simulink model "CSAD_Thrust_simulation"  (R2015a)
settings: Solver=ode3  StartTime=0.0  StopTime=350  FixedStep=0.01  MaxStep=10.0  RelTol=1e-3
values from neighbouring files (symbols this model uses):
  C = [C1;C2;C3]    [Spange_init.m]
  D = 3.0/100    (= 0.03)    [Spange_init.m]
  eps_c = 5    [Spange_init.m]
  epsilon = 0.5    [Spange_init.m]
  hd = c2d(H1,0.1,'foh')    [Spange_init.m]
  hd2 = c2d(H2,0.01,'zoh')    [Spange_init.m]
  I_s = 0.05    [Spange_init.m]
  k_cc = 1    [Spange_init.m]
  K_omega = 0.3    [Spange_init.m]
  K_q1f = 0.0113    [Spange_init.m]
  K_q1r = K_q1f    (= 0.0113)    [Spange_init.m]
  K_q2f = 0.0117    [Spange_init.m]
  K_q2r = K_q2f    (= 0.0117)    [Spange_init.m]
  K_q3f = 0.0113    [Spange_init.m]
  K_q3r = K_q3f    (= 0.0113)    [Spange_init.m]
  K_T1f = 0.3763    [Spange_init.m]
  K_T1r = K_T1f    (= 0.3763)    [Spange_init.m]
  K_T2f = 0.3901    [Spange_init.m]
  K_T2r = K_T2f    (= 0.3901)    [Spange_init.m]
  K_T3f = 0.3776    [Spange_init.m]
  K_T3r = K_T3f    (= 0.3776)    [Spange_init.m]
  Kp = 0.3    [Spange_init.m]
  Max_Acceleration = 2    [Spange_init.m]
  Max_rotation = 12*sqrt(lambda)    [Spange_init.m]
  Max_thrust = 1.5034    [Spange_init.m]
  Min_thrust = -0.85    [Spange_init.m]
  n_c = 5    [Spange_init.m]
  n_max = 64.6    [Spange_init.m]
  p_cc = 0.5    [Spange_init.m]
  Q_f0 = 0.3    [Spange_init.m]
  r_cc = 4    [Spange_init.m]
  Rho = Rho_m    (= 1000)    [Spange_init.m]
  tc = [u(1),u(2),u(3)]'    [Spange_thrustallocationQuadratic_mode1.m]    (also in Spange_thrustallocationQuadratic_mode2.m; Spange_thrustallocationQuadratic_mode3.m; Spange_thrustallocationQuadratic_mode4.m)
  Thruster_control = 1    [Spange_init.m]
undefined symbols (not defined in the file or in its folder): K_q4f, K_q4r, K_q5f, K_q5r, K_q6f, K_q6r, K_T4f, K_T4r, K_T5f, K_T5r, K_T6f, K_T6r, Thrust_algorithm, Thruster, Thruster_lock
libraries: simulink x6, simulink_extras x3
(part 1 of 2)
settings Model: CovModelRefEnable=off  Creator=Preben  LastModifiedBy=Preben
settings SolverCC: AlgebraicLoopSolver=LineSearch
settings DataIOCC: SaveFormat=Dataset
settings HardwareCC: ProdBitPerPointer=64  ProdLargestAtomicFloat=Float  ProdIntDivRoundTo=Zero  ProdEndianess=LittleEndian  ProdHWDeviceType=Specified

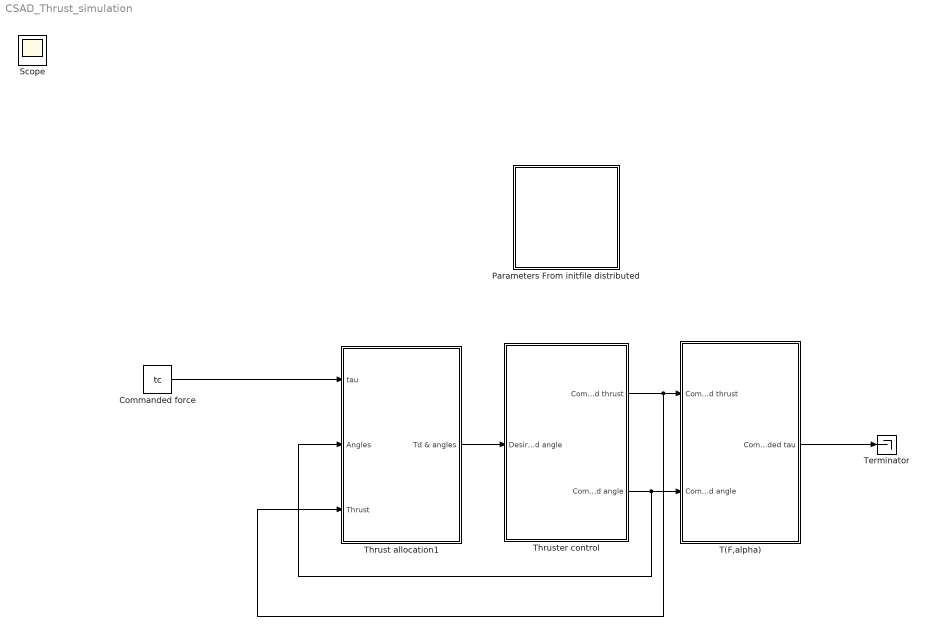
== system CSAD_Thrust_simulation ==
  Commanded force : Constant  Value=tc
  "Parameters From initfile distributed " : Subsystem
  T(F,alpha) : Subsystem
  Terminator : Terminator
  Thrust allocation1 : Subsystem
  "Thruster control " : Subsystem
  Scope : Scope
      settings: YMin=-10  YMax=10  SaveName=ScopeData2
  wires:
  "Thruster control "/2(Commanded angle) -> T(F,alpha)/2(Commanded angle), Thrust allocation1/2(Angles)
  Thrust allocation1/1(Td & angles) -> "Thruster control "/1("Desired thrust and angle ")
  "Thruster control "/1("Commanded thrust ") -> Thrust allocation1/3(Thrust), T(F,alpha)/1(Commanded thrust)
  T(F,alpha)/1(Commanded tau) -> Terminator/1
  Commanded force/1 -> Thrust allocation1/1(tau)

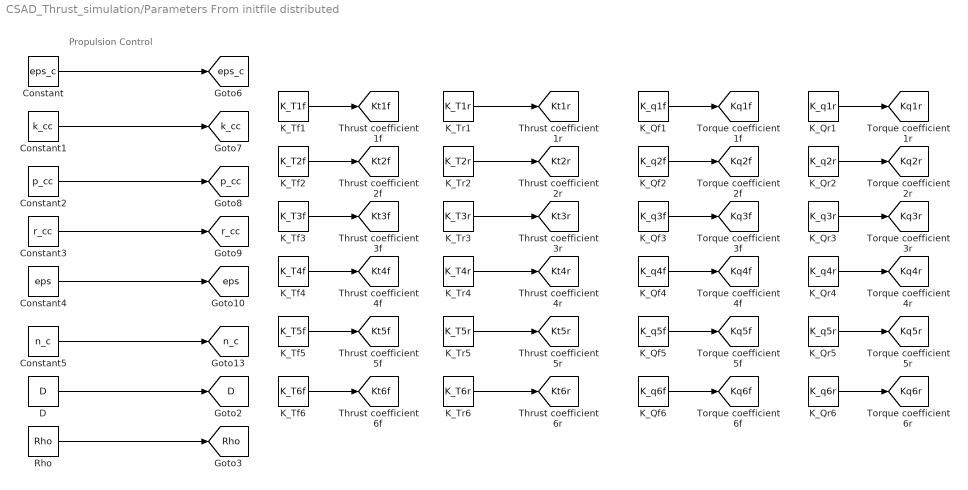
== system CSAD_Thrust_simulation/Parameters From initfile distributed  ==
  note: Propulsion Control
  Constant : Constant  Value=eps_c
  Constant1 : Constant  Value=k_cc
  Constant2 : Constant  Value=p_cc
  Constant3 : Constant  Value=r_cc
  Constant4 : Constant  Value=eps
  Constant5 : Constant  Value=n_c
  D : Constant  Value=D
  K_Qf1 : Constant  Value=K_q1f
  K_Qf2 : Constant  Value=K_q2f
  K_Qf3 : Constant  Value=K_q3f
  K_Qf4 : Constant  Value=K_q4f
  K_Qf5 : Constant  Value=K_q5f
  K_Qf6 : Constant  Value=K_q6f
  K_Qr1 : Constant  Value=K_q1r
  K_Qr2 : Constant  Value=K_q2r
  K_Qr3 : Constant  Value=K_q3r
  K_Qr4 : Constant  Value=K_q4r
  K_Qr5 : Constant  Value=K_q5r
  K_Qr6 : Constant  Value=K_q6r
  K_Tf1 : Constant  Value=K_T1f
  K_Tf2 : Constant  Value=K_T2f
  K_Tf3 : Constant  Value=K_T3f
  K_Tf4 : Constant  Value=K_T4f
  K_Tf5 : Constant  Value=K_T5f
  K_Tf6 : Constant  Value=K_T6f
  K_Tr1 : Constant  Value=K_T1r
  K_Tr2 : Constant  Value=K_T2r
  K_Tr3 : Constant  Value=K_T3r
  K_Tr4 : Constant  Value=K_T4r
  K_Tr5 : Constant  Value=K_T5r
  K_Tr6 : Constant  Value=K_T6r
  Rho : Constant  Value=Rho
  tag scope: D=global, Kq1f=global, Kq1r=global, Kq2f=global, Kq2r=global, Kq3f=global, Kq3r=global, Kq4f=global, Kq4r=global, Kq5f=global, Kq5r=global, Kq6f=global, Kq6r=global, Kt1f=global, Kt1r=global, Kt2f=global, Kt2r=global, Kt3f=global, Kt3r=global, Kt4f=global, Kt4r=global, Kt5f=global, Kt5r=global, Kt6f=global, Kt6r=global, Rho=global, eps=global, eps_c=global, k_cc=global, n_c=global, p_cc=global, r_cc=global
  wires:
  D/1 -> [D]
  Rho/1 -> [Rho]
  Constant/1 -> [eps_c]
  Constant1/1 -> [k_cc]
  Constant2/1 -> [p_cc]
  Constant3/1 -> [r_cc]
  Constant4/1 -> [eps]
  Constant5/1 -> [n_c]
  K_Tf1/1 -> [Kt1f]
  K_Tf6/1 -> [Kt6f]
  K_Tf5/1 -> [Kt5f]
  K_Tf4/1 -> [Kt4f]
  K_Tf3/1 -> [Kt3f]
  K_Tf2/1 -> [Kt2f]
  K_Tr1/1 -> [Kt1r]
  K_Tr6/1 -> [Kt6r]
  K_Tr5/1 -> [Kt5r]
  K_Tr4/1 -> [Kt4r]
  K_Tr2/1 -> [Kt2r]
  K_Tr3/1 -> [Kt3r]
  K_Qf1/1 -> [Kq1f]
  K_Qf2/1 -> [Kq2f]
  K_Qf3/1 -> [Kq3f]
  K_Qf4/1 -> [Kq4f]
  K_Qf5/1 -> [Kq5f]
  K_Qf6/1 -> [Kq6f]
  K_Qr1/1 -> [Kq1r]
  K_Qr2/1 -> [Kq2r]
  K_Qr3/1 -> [Kq3r]
  K_Qr4/1 -> [Kq4r]
  K_Qr5/1 -> [Kq5r]
  K_Qr6/1 -> [Kq6r]

== system CSAD_Thrust_simulation/T(F,alpha) ==
  Commanded thrust : Inport
  Commanded angle : Inport  Port=2
  MATLAB Function : MATLAB Function  TreatAsAtomicUnit=on
  Radians to Degrees : simulink_extras/Transformations/Radians to Degrees
  X-position Thruster : Constant  Value=[Thruster.T1(1) Thruster.T2(1) Thruster.T3(1) Thruster.T4(1) Thruster.T5(1) Thruster.T6(1)]
  Y-position Thruster : Constant  Value=[Thruster.T1(2) Thruster.T2(2) Thruster.T3(2) Thruster.T4(2) Thruster.T5(2) Thruster.T6(2)]
  Commanded tau : Outport
  wires:
  Commanded angle/1 -> Radians to Degrees/1
  X-position Thruster/1 -> MATLAB Function/3(PosX)
  Y-position Thruster/1 -> MATLAB Function/4(PosY)
  MATLAB Function/1(actual_tau) -> Commanded tau/1
  Commanded thrust/1 -> MATLAB Function/1(thrust_actual)
  Radians to Degrees/1 -> MATLAB Function/2(alpha_actual)

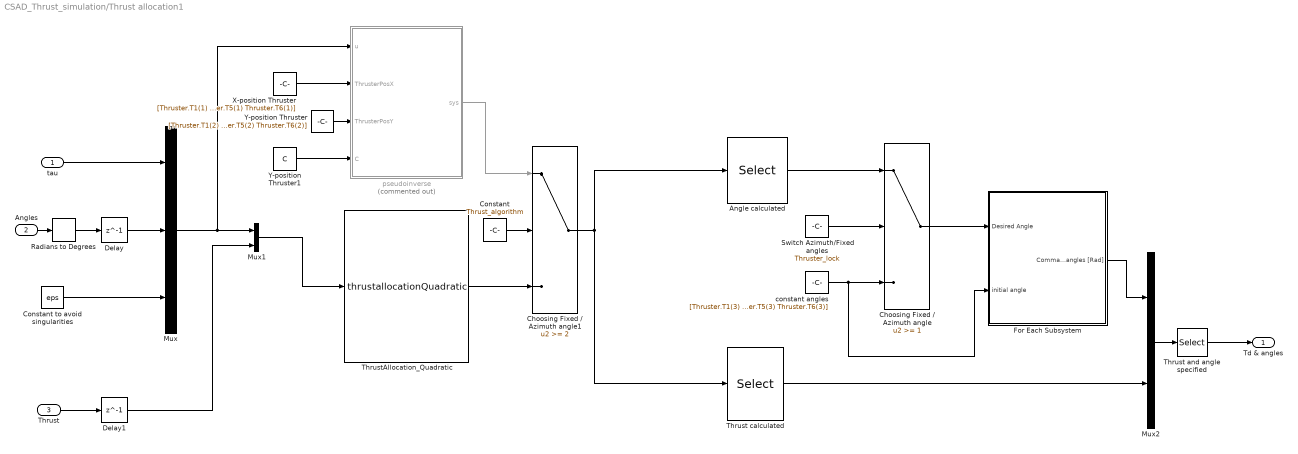
== system CSAD_Thrust_simulation/Thrust allocation1 ==
  tau : Inport
  Angles : Inport  Port=2
  Thrust : Inport  Port=3
  "  Thrust calculated" : Selector  InputPortWidth=12  Indices=[7 8 9 10 11 12]
  " Angle calculated" : Selector  InputPortWidth=12  Indices=[1 2 3 4 5 6]
  Choosing Fixed / Azimuth angle : Switch  Threshold=1
  Choosing Fixed / Azimuth angle1 : Switch  Threshold=2
  Constant : Constant  Value=Thrust_algorithm
  Constant to avoid singularities : Constant  Value=eps
  Delay : Delay  DelayLength=1  InitialCondition=0
  Delay1 : Delay  DelayLength=1  InitialCondition=0
  For Each Subsystem : Subsystem  TreatAsAtomicUnit=on
  Mux : Mux  Inputs=3
  Mux1 : Mux  Inputs=2
  Mux2 : Mux  Inputs=2
  Radians to Degrees : simulink_extras/Transformations/Radians to Degrees
  Switch Azimuth/Fixed angles : Constant  Value=Thruster_lock
  Thrust and angle specified : Selector  InputPortWidth=12  Indices=[7 1 8 2 9 3 10 4 11 5 12 6]
  ThrustAllocation_Quadratic : S-Function  RequirementInfo={} %GIDa_b0499093_94a1_4fb6_935a_9715d93fd690  FunctionName=thrustallocationQuadratic  Parameters=Thruster,C
  X-position Thruster : Constant  Value=[Thruster.T1(1) Thruster.T2(1) Thruster.T3(1) Thruster.T4(1) Thruster.T5(1) Thruster.T6(1)]
  Y-position Thruster : Constant  Value=[Thruster.T1(2) Thruster.T2(2) Thruster.T3(2) Thruster.T4(2) Thruster.T5(2) Thruster.T6(2)]
  Y-position Thruster1 : Constant  Value=C
  constant angles : Constant  Value=[Thruster.T1(3) Thruster.T2(3) Thruster.T3(3) Thruster.T4(3) Thruster.T5(3) Thruster.T6(3)]
  pseudoinverse : MATLAB Function  Commented=on  TreatAsAtomicUnit=on
  Td & angles : Outport
  wires:
  Switch Azimuth/Fixed angles/1 -> Choosing Fixed / Azimuth angle/2
  Constant to avoid singularities/1 -> Mux/3
  " Angle calculated"/1 -> Choosing Fixed / Azimuth angle/1
  Thrust and angle specified/1 -> Td & angles/1
  Mux2/1 -> Thrust and angle specified/1
  tau/1 -> Mux/1
  Choosing Fixed / Azimuth angle/1 -> For Each Subsystem/1(Desired Angle)
  Angles/1 -> Radians to Degrees/1
  For Each Subsystem/1("Commanded angles [Rad] ") -> Mux2/1
  constant angles/1 -> For Each Subsystem/2("initial angle "), Choosing Fixed / Azimuth angle/3
  Radians to Degrees/1 -> Delay/1
  Mux1/1 -> ThrustAllocation_Quadratic/1
  Thrust/1 -> Delay1/1
  "  Thrust calculated"/1 -> Mux2/2
  Delay/1 -> Mux/2
  Delay1/1 -> Mux1/2
  Choosing Fixed / Azimuth angle1/1 -> " Angle calculated"/1, "  Thrust calculated"/1
  Mux/1 -> pseudoinverse/1(u), Mux1/1
  X-position Thruster/1 -> pseudoinverse/2(ThrusterPosX)
  Y-position Thruster/1 -> pseudoinverse/3(ThrusterPosY)
  Y-position Thruster1/1 -> pseudoinverse/4(C)
  ThrustAllocation_Quadratic/1 -> Choosing Fixed / Azimuth angle1/3
  pseudoinverse/1(sys) -> Choosing Fixed / Azimuth angle1/1
  Constant/1 -> Choosing Fixed / Azimuth angle1/2

== system CSAD_Thrust_simulation/Thruster control  ==
  "Desired thrust and angle " : Inport
  Demux : Demux  Outputs=12
  Mux : Mux  Inputs=12
  Selecting Actual thrust : Selector  InputPortWidth=12  Indices=[1 3 5 7 9 11]
  Selecting actual angle : Selector  InputPortWidth=12  Indices=[2 4 6 8 10 12]
  Subsystem : Subsystem
  Thruster 1 : Subsystem
      settings: AttributesFormatString=%<MinAlgLoopOccurrences>
  Thruster 2 : Subsystem
      settings: AttributesFormatString=%<MinAlgLoopOccurrences>
  Thruster 3 : Subsystem
      settings: AttributesFormatString=%<MinAlgLoopOccurrences>
  Thruster 4 : Subsystem
      settings: AttributesFormatString=%<MinAlgLoopOccurrences>
  Thruster 5 : Subsystem
      settings: AttributesFormatString=%<MinAlgLoopOccurrences>
  Thruster 6 : Subsystem
      settings: AttributesFormatString=%<MinAlgLoopOccurrences>
  "Commanded thrust " : Outport
  Commanded angle : Outport  Port=2
  wires:
  "Desired thrust and angle "/1 -> Demux/1
  Demux/3 -> Thruster 2/1(Desired thrust 1)
  Demux/4 -> Thruster 2/2(Desired Angle)
  Demux/5 -> Thruster 3/1(Desired thrust 1)
  Demux/6 -> Thruster 3/2(Desired Angle)
  Demux/7 -> Thruster 4/1(Desired thrust 1)
  Demux/8 -> Thruster 4/2(Desired Angle)
  Demux/9 -> Thruster 5/1(Desired thrust 1)
  Demux/10 -> Thruster 5/2(Desired Angle)
  Demux/11 -> Thruster 6/1(Desired thrust 1)
  Demux/12 -> Thruster 6/2(Desired Angle)
  Thruster 1/1(Commanded thrust 1) -> Mux/1
  Thruster 2/1(Commanded thrust 1) -> Mux/3
  Thruster 2/2(Commanded angle) -> Mux/4
  Thruster 3/1("Commanded thrust ") -> Mux/5
  Thruster 3/2(Commanded angle) -> Mux/6
  Thruster 4/1("Commanded thrust ") -> Mux/7
  Thruster 4/2(Commanded angle) -> Mux/8
  Thruster 5/1(Commanded thrust 1) -> Mux/9
  Thruster 5/2(Commanded angle) -> Mux/10
  Thruster 6/1(Commanded thrust 1) -> Mux/11
  Thruster 6/2(Commanded angle) -> Mux/12
  Mux/1 -> Selecting Actual thrust/1, Selecting actual angle/1
  Demux/2 -> Thruster 1/2(Desired Angle)
  Thruster 1/2(Commanded angle) -> Mux/2
  Selecting actual angle/1 -> Commanded angle/1
  Subsystem/1(Thrust from model) -> "Commanded thrust "/1
  Selecting Actual thrust/1 -> Subsystem/1(Calculated thrust)
  Demux/1 -> Thruster 1/1(Desired thrust 1)

== system CSAD_Thrust_simulation/Thrust allocation1/For Each Subsystem ==
  Desired Angle : Inport  Partition=on  PartitionDimension=1  PartitionWidth=1
  "initial angle " : Inport  Port=2  Partition=on  PartitionDimension=1  PartitionWidth=1
  Degrees to Radians : simulink_extras/Transformations/Degrees to Radians
  Ensures fastest way is chosen : MATLAB Function  TreatAsAtomicUnit=on
  For Each : ForEach  DisableCoverage=on  IndexMode=One-based
  Integrator : Integrator  ExternalReset=either  InitialConditionSource=external
  MATLAB Function : MATLAB Function  TreatAsAtomicUnit=on
  Max Rotation Rate : Saturate  UpperLimit=Max_rotation  LowerLimit=-Max_rotation
  constant : Constant  Value=0
  "Commanded angles [Rad] " : Outport  ConcatenationDimension=1
  wires:
  Degrees to Radians/1 -> MATLAB Function/1(angle)
  MATLAB Function/1(y) -> "Commanded angles [Rad] "/1
  Integrator/1 -> Degrees to Radians/1, Ensures fastest way is chosen/2(actual)  "angle"
  "initial angle "/1 -> Integrator/3
  Max Rotation Rate/1 -> Integrator/1
  Ensures fastest way is chosen/1(psi_D) -> Max Rotation Rate/1
  Desired Angle/1 -> Ensures fastest way is chosen/1(desired)
  constant/1 -> Integrator/2

== system CSAD_Thrust_simulation/Thruster control /Subsystem ==
  Calculated thrust : Inport
  Demux : Demux  Outputs=6
  Mux : Mux  Inputs=6
  Saturation {1..6} (6 alike) : Saturate  UpperLimit=Max_thrust  LowerLimit=Min_thrust
  Thrust from model : Outport
  wires:
  Calculated thrust/1 -> Demux/1
  Demux/1 -> Saturation 1/1
  Demux/2 -> Saturation 2/1
  Demux/3 -> Saturation 3/1
  Demux/4 -> Saturation 4/1
  Demux/5 -> Saturation 5/1
  Demux/6 -> Saturation 6/1
  Mux/1 -> Thrust from model/1
  Saturation 1/1 -> Mux/1
  Saturation 6/1 -> Mux/6
  Saturation 5/1 -> Mux/5
  Saturation 4/1 -> Mux/4
  Saturation 3/1 -> Mux/3
  Saturation 2/1 -> Mux/2

== system CSAD_Thrust_simulation/Thruster control /Thruster 1 ==
  Desired thrust 1 : Inport
  Desired Angle : Inport  Port=2
  Constant : Constant  Value=hd2.den{1,1}
  Constant1 : Constant  Value=hd2.num{1,1}
  Discrete Transfer Fcn : DiscreteTransferFcn  NumeratorSource=Input port  DenominatorSource=Input port  Denominator=[0.2 1]  SampleTime=0.01  a0EqualsOne=on
      settings: InputPortMap=u0,p1,p3
  Losses (placeholder) : Constant  Value=0
  Propeller Hydrodynamics : Subsystem
  Shaft dynamics : Subsystem
  Thruster control : Subsystem
  Commanded thrust 1 : Outport
  Commanded angle : Outport  Port=2
  wires:
  Losses (placeholder)/1 -> Propeller Hydrodynamics/1(env)
  Propeller Hydrodynamics/1(Ta) -> Commanded thrust 1/1
  Thruster control/1(Qc) -> Discrete Transfer Fcn/1
  Desired Angle/1 -> Commanded angle/1
  Constant1/1 -> Discrete Transfer Fcn/2
  Constant/1 -> Discrete Transfer Fcn/3
  Shaft dynamics/1(n) -> Thruster control/2(n), Propeller Hydrodynamics/2(n)
  Propeller Hydrodynamics/2(Qa) -> Shaft dynamics/2(Qa)
  Discrete Transfer Fcn/1 -> Shaft dynamics/1(Qm)
  Desired thrust 1/1 -> Thruster control/1("T_d ")

== system CSAD_Thrust_simulation/Thruster control /Thruster 2 ==
  Desired thrust 1 : Inport
  Desired Angle : Inport  Port=2
  Constant : Constant  Value=hd2.den{1,1}
  Constant1 : Constant  Value=hd2.num{1,1}
  Discrete Transfer Fcn : DiscreteTransferFcn  NumeratorSource=Input port  DenominatorSource=Input port  Denominator=[0.2 1]  SampleTime=0.01  a0EqualsOne=on
      settings: InputPortMap=u0,p1,p3
  Losses (placeholder) : Constant  Value=0
  Propeller Hydrodynamics : Subsystem
  Shaft dynamics : Subsystem
  Thruster control : Subsystem
  Commanded thrust 1 : Outport
  Commanded angle : Outport  Port=2
  wires:
  Losses (placeholder)/1 -> Propeller Hydrodynamics/1(env)
  Thruster control/1(Qc) -> Discrete Transfer Fcn/1
  Discrete Transfer Fcn/1 -> Shaft dynamics/1(Qm)
  Desired thrust 1/1 -> Thruster control/1("T_d ")
  Propeller Hydrodynamics/1(Ta) -> Commanded thrust 1/1
  Desired Angle/1 -> Commanded angle/1
  Constant1/1 -> Discrete Transfer Fcn/2
  Constant/1 -> Discrete Transfer Fcn/3
  Shaft dynamics/1(n) -> Thruster control/2(n), Propeller Hydrodynamics/2(n)
  Propeller Hydrodynamics/2(Qa) -> Shaft dynamics/2(Qa)

== system CSAD_Thrust_simulation/Thruster control /Thruster 3 ==
  Desired thrust 1 : Inport
  Desired Angle : Inport  Port=2
  Constant : Constant  Value=hd2.den{1,1}
  Constant1 : Constant  Value=hd2.num{1,1}
  Discrete Transfer Fcn : DiscreteTransferFcn  NumeratorSource=Input port  DenominatorSource=Input port  Denominator=[0.2 1]  SampleTime=0.01  a0EqualsOne=on
      settings: InputPortMap=u0,p1,p3
  Losses (placeholder) : Constant  Value=0
  Propeller Hydrodynamics : Subsystem
  Shaft dynamics : Subsystem
  Thruster control : Subsystem
  "Commanded thrust " : Outport
  Commanded angle : Outport  Port=2
  wires:
  Losses (placeholder)/1 -> Propeller Hydrodynamics/1(env)
  Thruster control/1(Qc) -> Discrete Transfer Fcn/1
  Discrete Transfer Fcn/1 -> Shaft dynamics/1(Qm)
  Desired thrust 1/1 -> Thruster control/1("T_d ")
  Propeller Hydrodynamics/1(Ta) -> "Commanded thrust "/1
  Desired Angle/1 -> Commanded angle/1
  Constant1/1 -> Discrete Transfer Fcn/2
  Constant/1 -> Discrete Transfer Fcn/3
  Shaft dynamics/1(n) -> Thruster control/2(n), Propeller Hydrodynamics/2(n)
  Propeller Hydrodynamics/2(Qa) -> Shaft dynamics/2(Qa)

== system CSAD_Thrust_simulation/Thruster control /Thruster 4 ==
  Desired thrust 1 : Inport
  Desired Angle : Inport  Port=2
  Constant : Constant  Value=hd2.den{1,1}
  Constant1 : Constant  Value=hd2.num{1,1}
  Discrete Transfer Fcn : DiscreteTransferFcn  NumeratorSource=Input port  DenominatorSource=Input port  Denominator=[0.2 1]  SampleTime=0.01  a0EqualsOne=on
      settings: InputPortMap=u0,p1,p3
  Losses (placeholder) : Constant  Value=0
  Propeller Hydrodynamics : Subsystem
  Shaft dynamics : Subsystem
  Thruster control : Subsystem
  "Commanded thrust " : Outport
  Commanded angle : Outport  Port=2
  wires:
  Losses (placeholder)/1 -> Propeller Hydrodynamics/1(env)
  Thruster control/1(Qc) -> Discrete Transfer Fcn/1
  Discrete Transfer Fcn/1 -> Shaft dynamics/1(Qm)
  Desired thrust 1/1 -> Thruster control/1("T_d ")
  Propeller Hydrodynamics/1(Ta) -> "Commanded thrust "/1
  Desired Angle/1 -> Commanded angle/1
  Constant1/1 -> Discrete Transfer Fcn/2
  Constant/1 -> Discrete Transfer Fcn/3
  Shaft dynamics/1(n) -> Thruster control/2(n), Propeller Hydrodynamics/2(n)
  Propeller Hydrodynamics/2(Qa) -> Shaft dynamics/2(Qa)

== system CSAD_Thrust_simulation/Thruster control /Thruster 5 ==
  Desired thrust 1 : Inport
  Desired Angle : Inport  Port=2
  Constant : Constant  Value=hd2.den{1,1}
  Constant1 : Constant  Value=hd2.num{1,1}
  Discrete Transfer Fcn : DiscreteTransferFcn  NumeratorSource=Input port  DenominatorSource=Input port  Denominator=[0.2 1]  SampleTime=0.01  a0EqualsOne=on
      settings: InputPortMap=u0,p1,p3
  Losses (placeholder) : Constant  Value=0
  Propeller Hydrodynamics : Subsystem
  Shaft dynamics : Subsystem
  Thruster control : Subsystem
  Commanded thrust 1 : Outport
  Commanded angle : Outport  Port=2
  wires:
  Losses (placeholder)/1 -> Propeller Hydrodynamics/1(env)
  Thruster control/1(Qc) -> Discrete Transfer Fcn/1
  Discrete Transfer Fcn/1 -> Shaft dynamics/1(Qm)
  Desired thrust 1/1 -> Thruster control/1("T_d ")
  Propeller Hydrodynamics/1(Ta) -> Commanded thrust 1/1
  Desired Angle/1 -> Commanded angle/1
  Constant1/1 -> Discrete Transfer Fcn/2
  Constant/1 -> Discrete Transfer Fcn/3
  Shaft dynamics/1(n) -> Thruster control/2(n), Propeller Hydrodynamics/2(n)
  Propeller Hydrodynamics/2(Qa) -> Shaft dynamics/2(Qa)

== system CSAD_Thrust_simulation/Thruster control /Thruster 6 ==
  Desired thrust 1 : Inport
  Desired Angle : Inport  Port=2
  Constant : Constant  Value=hd2.den{1,1}
  Constant1 : Constant  Value=hd2.num{1,1}
  Discrete Transfer Fcn : DiscreteTransferFcn  NumeratorSource=Input port  DenominatorSource=Input port  Denominator=[0.2 1]  SampleTime=0.01  a0EqualsOne=on
      settings: InputPortMap=u0,p1,p3
  Losses (placeholder) : Constant  Value=0
  Propeller Hydrodynamics : Subsystem
  Shaft dynamics : Subsystem
  Thruster control : Subsystem
  Commanded thrust 1 : Outport
  Commanded angle : Outport  Port=2
  wires:
  Losses (placeholder)/1 -> Propeller Hydrodynamics/1(env)
  Thruster control/1(Qc) -> Discrete Transfer Fcn/1
  Discrete Transfer Fcn/1 -> Shaft dynamics/1(Qm)
  Desired thrust 1/1 -> Thruster control/1("T_d ")
  Propeller Hydrodynamics/1(Ta) -> Commanded thrust 1/1
  Desired Angle/1 -> Commanded angle/1
  Constant1/1 -> Discrete Transfer Fcn/2
  Constant/1 -> Discrete Transfer Fcn/3
  Propeller Hydrodynamics/2(Qa) -> Shaft dynamics/2(Qa)
  Shaft dynamics/1(n) -> Thruster control/2(n), Propeller Hydrodynamics/2(n)

== system CSAD_Thrust_simulation/Thruster control /Thruster 1/Propeller Hydrodynamics ==
  env : Inport
  n : Inport  Port=2
  Actual Force and Torque : MATLAB Function  TreatAsAtomicUnit=on
  Ta : Outport
  Qa : Outport  Port=2
  wires:
  n/1 -> Actual Force and Torque/1(n)
  [D] -> Actual Force and Torque/7(D)
  [Kq1f] -> Actual Force and Torque/2(Kq)
  Actual Force and Torque/2(Qa) -> Qa/1
  [Rho] -> Actual Force and Torque/6(Rho)
  env/1 -> Actual Force and Torque/9(env)
  [Kt1f] -> Actual Force and Torque/3(Kt)
  Actual Force and Torque/1(Ta) -> Ta/1
  [Kt1r] -> Actual Force and Torque/4(Ktr)
  [Kq1r] -> Actual Force and Torque/5(Kqr)
  [eps_c] -> Actual Force and Torque/8(eps_c)

== system CSAD_Thrust_simulation/Thruster control /Thruster 1/Shaft dynamics ==
  Qm : Inport
  Qa : Inport  Port=2
  Constant : Constant  Value=0
  Finding rotation speed : Gain  Gain=1/(2*pi*I_s)
  Integrator : Integrator  ExternalReset=either
  K_omega : Gain  Gain=K_omega*2*pi
  Sum : Sum  Inputs=-+-
  n : Outport
  wires:
  Qm/1 -> Sum/2
  Sum/1 -> Finding rotation speed/1
  Qa/1 -> Sum/1
  K_omega/1 -> Sum/3
  Finding rotation speed/1 -> Integrator/1
  Integrator/1 -> n/1, K_omega/1
  Constant/1 -> Integrator/2

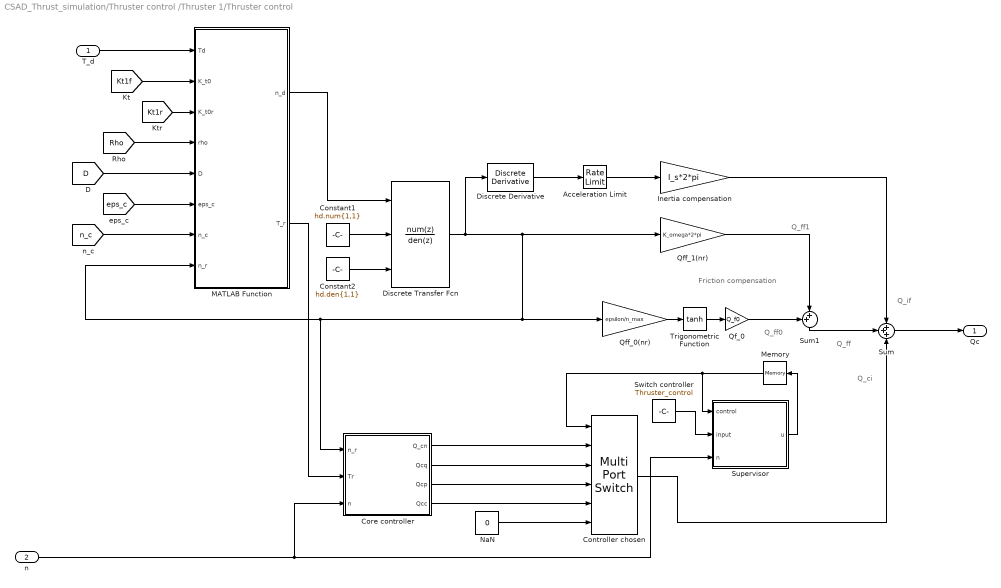
== system CSAD_Thrust_simulation/Thruster control /Thruster 1/Thruster control ==
  note: Q_ci
  note: Q_if
  note: Q_ff
  note: Q_ff0
  note: Q_ff1
  note: Friction compensation
  "T_d " : Inport
  n : Inport  Port=2
  Acceleration Limit : RateLimiter  RisingSlewLimit=Max_Acceleration  FallingSlewLimit=-Max_Acceleration  SampleTimeMode=inherited
  Constant1 : Constant  Value=hd.num{1,1}  VectorParams1D=off
  Constant2 : Constant  Value=hd.den{1,1}  VectorParams1D=off
  Controller chosen : MultiPortSwitch  Inputs=5
  Core controller : Subsystem
  Discrete Transfer Fcn : DiscreteTransferFcn  NumeratorSource=Input port  Numerator=[8.76e-05 0.0003481 8.648e-05]  DenominatorSource=Input port  Denominator=[1 -1.974 0.9746]  SampleTime=0.01  a0EqualsOne=on
      settings: InputPortMap=u0,p1,p3
  Discrete Derivative : simulink/Discrete/Discrete Derivative  gainval=1.0  ICPrevScaledInput=0.0  InputProcessing=Inherited  OutMin=[]  OutMax=[]  OutDataType=fixdt(1, 16)  OutScaling=2^-10  DoSatur=off
  Inertia compensation : Gain  Gain=I_s*2*pi
  MATLAB Function : MATLAB Function  TreatAsAtomicUnit=on
  Memory : Memory  X0=1  InheritSampleTime=on
  NaN : Constant  Value=0
  Qf_0 : Gain  Gain=Q_f0
  Qff_0(nr) : Gain  Gain=epsilon/n_max
  Qff_1(nr) : Gain  Gain=K_omega*2*pi
  Sum : Sum  Inputs=+++
  Sum1 : Sum  Inputs=++|
  Supervisor : MATLAB Function  TreatAsAtomicUnit=on
  Switch controller : Constant  Value=Thruster_control
  Trigonometric Function : Trigonometry  Operator=tanh
  Qc : Outport
  wires:
  [Rho] -> MATLAB Function/4(rho)
  [D] -> MATLAB Function/5(D)
  [eps_c] -> MATLAB Function/6(eps_c)
  MATLAB Function/2(T_r) -> Core controller/2("Tr ")
  MATLAB Function/1(n_d) -> Discrete Transfer Fcn/1
  Qff_0(nr)/1 -> Trigonometric Function/1
  Trigonometric Function/1 -> Qf_0/1
  NaN/1 -> Controller chosen/6
  Supervisor/1(u) -> Memory/1
  Memory/1 -> Controller chosen/1, Supervisor/1(control)
  Qff_1(nr)/1 -> Sum1/2
  Qf_0/1 -> Sum1/1
  Switch controller/1 -> Supervisor/2(input)
  Controller chosen/1 -> Sum/3
  Core controller/2(Qcq) -> Controller chosen/3
  Core controller/3(Qcp) -> Controller chosen/4
  Core controller/4(Qcc) -> Controller chosen/5
  Core controller/1(Q_cn) -> Controller chosen/2
  [n_c] -> MATLAB Function/7(n_c)
  Discrete Derivative/1 -> Acceleration Limit/1
  Sum1/1 -> Sum/2
  Constant1/1 -> Discrete Transfer Fcn/2
  Constant2/1 -> Discrete Transfer Fcn/3
  Inertia compensation/1 -> Sum/1
  n/1 -> Core controller/3("n "), Supervisor/3(n)
  Acceleration Limit/1 -> Inertia compensation/1
  Discrete Transfer Fcn/1 -> Core controller/1(n_r), MATLAB Function/8(n_r), Qff_0(nr)/1, Qff_1(nr)/1, Discrete Derivative/1
  "T_d "/1 -> MATLAB Function/1(Td)
  [Kt1f] -> MATLAB Function/2(K_t0)
  [Kt1r] -> MATLAB Function/3(K_t0r)
  Sum/1 -> Qc/1

== system CSAD_Thrust_simulation/Thruster control /Thruster 2/Propeller Hydrodynamics ==
  env : Inport
  n : Inport  Port=2
  Actual Force and Torque : MATLAB Function  TreatAsAtomicUnit=on
  Ta : Outport
  Qa : Outport  Port=2
  wires:
  n/1 -> Actual Force and Torque/1(n)
  [D] -> Actual Force and Torque/7(D)
  [Kq2f] -> Actual Force and Torque/2(Kq)
  Actual Force and Torque/2(Qa) -> Qa/1
  [Rho] -> Actual Force and Torque/6(Rho)
  env/1 -> Actual Force and Torque/9(env)
  [Kt2f] -> Actual Force and Torque/3(Kt)
  Actual Force and Torque/1(Ta) -> Ta/1
  [Kt2r] -> Actual Force and Torque/4(Ktr)
  [Kq2r] -> Actual Force and Torque/5(Kqr)
  [eps_c] -> Actual Force and Torque/8(eps_c)

== system CSAD_Thrust_simulation/Thruster control /Thruster 2/Shaft dynamics ==
  Qm : Inport
  Qa : Inport  Port=2
  Constant : Constant  Value=0
  Finding rotation speed : Gain  Gain=1/(2*pi*I_s)
  Integrator : Integrator  ExternalReset=either
  K_omega : Gain  Gain=K_omega*2*pi
  Sum : Sum  Inputs=-+-
  n : Outport
  wires:
  Qm/1 -> Sum/2
  Sum/1 -> Finding rotation speed/1
  Qa/1 -> Sum/1
  K_omega/1 -> Sum/3
  Finding rotation speed/1 -> Integrator/1
  Integrator/1 -> K_omega/1, n/1
  Constant/1 -> Integrator/2

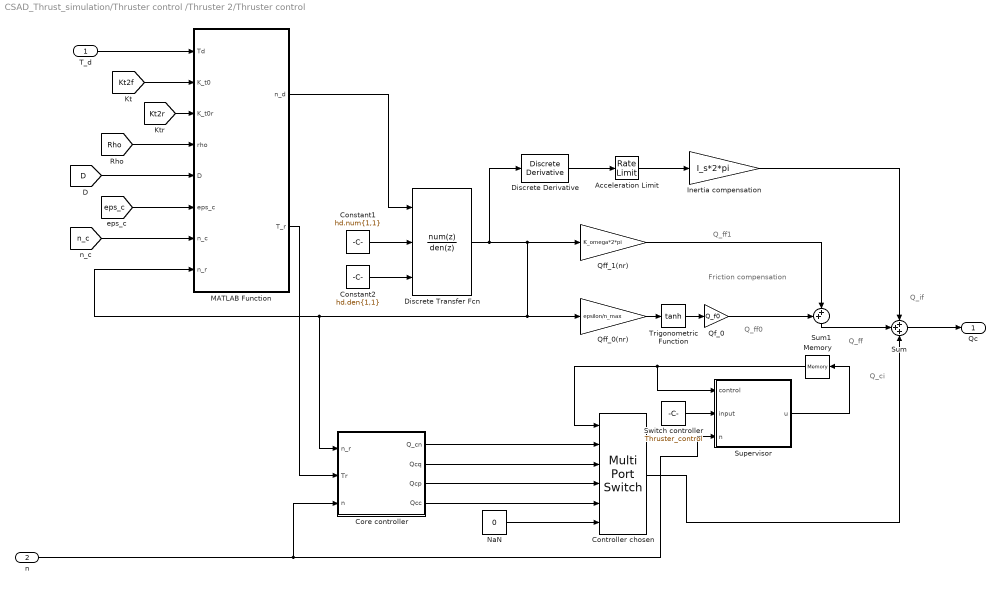
== system CSAD_Thrust_simulation/Thruster control /Thruster 2/Thruster control ==
  note: Q_ci
  note: Q_if
  note: Q_ff
  note: Q_ff0
  note: Q_ff1
  note: Friction compensation
  "T_d " : Inport
  n : Inport  Port=2
  Acceleration Limit : RateLimiter  RisingSlewLimit=Max_Acceleration  FallingSlewLimit=-Max_Acceleration  SampleTimeMode=inherited
  Constant1 : Constant  Value=hd.num{1,1}  VectorParams1D=off
  Constant2 : Constant  Value=hd.den{1,1}  VectorParams1D=off
  Controller chosen : MultiPortSwitch  Inputs=5
  Core controller : Subsystem
  Discrete Transfer Fcn : DiscreteTransferFcn  NumeratorSource=Input port  Numerator=[8.76e-05 0.0003481 8.648e-05]  DenominatorSource=Input port  Denominator=[1 -1.974 0.9746]  SampleTime=0.01  a0EqualsOne=on
      settings: InputPortMap=u0,p1,p3
  Discrete Derivative : simulink/Discrete/Discrete Derivative  gainval=1.0  ICPrevScaledInput=0.0  InputProcessing=Inherited  OutMin=[]  OutMax=[]  OutDataType=fixdt(1, 16)  OutScaling=2^-10  DoSatur=off
  Inertia compensation : Gain  Gain=I_s*2*pi
  MATLAB Function : MATLAB Function  TreatAsAtomicUnit=on
  Memory : Memory  X0=1
  NaN : Constant  Value=0
  Qf_0 : Gain  Gain=Q_f0
  Qff_0(nr) : Gain  Gain=epsilon/n_max
  Qff_1(nr) : Gain  Gain=K_omega*2*pi
  Sum : Sum  Inputs=+++
  Sum1 : Sum  Inputs=++|
  Supervisor : MATLAB Function  TreatAsAtomicUnit=on
  Switch controller : Constant  Value=Thruster_control
  Trigonometric Function : Trigonometry  Operator=tanh
  Qc : Outport
  wires:
  MATLAB Function/2(T_r) -> Core controller/2("Tr ")
  Qff_0(nr)/1 -> Trigonometric Function/1
  Trigonometric Function/1 -> Qf_0/1
  Sum1/1 -> Sum/2
  Core controller/1(Q_cn) -> Controller chosen/2
  Core controller/4(Qcc) -> Controller chosen/5
  NaN/1 -> Controller chosen/6
  Supervisor/1(u) -> Memory/1
  Memory/1 -> Supervisor/1(control), Controller chosen/1
  Qff_1(nr)/1 -> Sum1/2
  Qf_0/1 -> Sum1/1
  Controller chosen/1 -> Sum/3
  Inertia compensation/1 -> Sum/1
  Core controller/3(Qcp) -> Controller chosen/4
  Core controller/2(Qcq) -> Controller chosen/3
  Switch controller/1 -> Supervisor/2(input)
  "T_d "/1 -> MATLAB Function/1(Td)
  [Rho] -> MATLAB Function/4(rho)
  [D] -> MATLAB Function/5(D)
  [eps_c] -> MATLAB Function/6(eps_c)
  [n_c] -> MATLAB Function/7(n_c)
  Constant1/1 -> Discrete Transfer Fcn/2
  Constant2/1 -> Discrete Transfer Fcn/3
  MATLAB Function/1(n_d) -> Discrete Transfer Fcn/1
  Discrete Derivative/1 -> Acceleration Limit/1
  n/1 -> Core controller/3("n "), Supervisor/3(n)
  Acceleration Limit/1 -> Inertia compensation/1
  Discrete Transfer Fcn/1 -> Discrete Derivative/1, Qff_0(nr)/1, MATLAB Function/8(n_r), Core controller/1(n_r), Qff_1(nr)/1
  Sum/1 -> Qc/1
  [Kt2f] -> MATLAB Function/2(K_t0)
  [Kt2r] -> MATLAB Function/3(K_t0r)

== system CSAD_Thrust_simulation/Thruster control /Thruster 3/Propeller Hydrodynamics ==
  env : Inport
  n : Inport  Port=2
  Actual Force and Torque : MATLAB Function  TreatAsAtomicUnit=on
  Ta : Outport
  Qa : Outport  Port=2
  wires:
  n/1 -> Actual Force and Torque/1(n)
  [D] -> Actual Force and Torque/7(D)
  [Kq3f] -> Actual Force and Torque/2(Kq)
  Actual Force and Torque/2(Qa) -> Qa/1
  [Rho] -> Actual Force and Torque/6(Rho)
  env/1 -> Actual Force and Torque/9(env)
  [Kt3f] -> Actual Force and Torque/3(Kt)
  Actual Force and Torque/1(Ta) -> Ta/1
  [Kt3r] -> Actual Force and Torque/4(Ktr)
  [Kq3r] -> Actual Force and Torque/5(Kqr)
  [eps_c] -> Actual Force and Torque/8(eps_c)

== system CSAD_Thrust_simulation/Thruster control /Thruster 3/Shaft dynamics ==
  Qm : Inport
  Qa : Inport  Port=2
  Constant : Constant  Value=0
  Finding rotation speed : Gain  Gain=1/(2*pi*I_s)
  Integrator : Integrator  ExternalReset=either
  K_omega : Gain  Gain=K_omega*2*pi
  Sum : Sum  Inputs=-+-
  n : Outport
  wires:
  Qm/1 -> Sum/2
  Sum/1 -> Finding rotation speed/1
  Qa/1 -> Sum/1
  K_omega/1 -> Sum/3
  Finding rotation speed/1 -> Integrator/1
  Integrator/1 -> n/1, K_omega/1
  Constant/1 -> Integrator/2

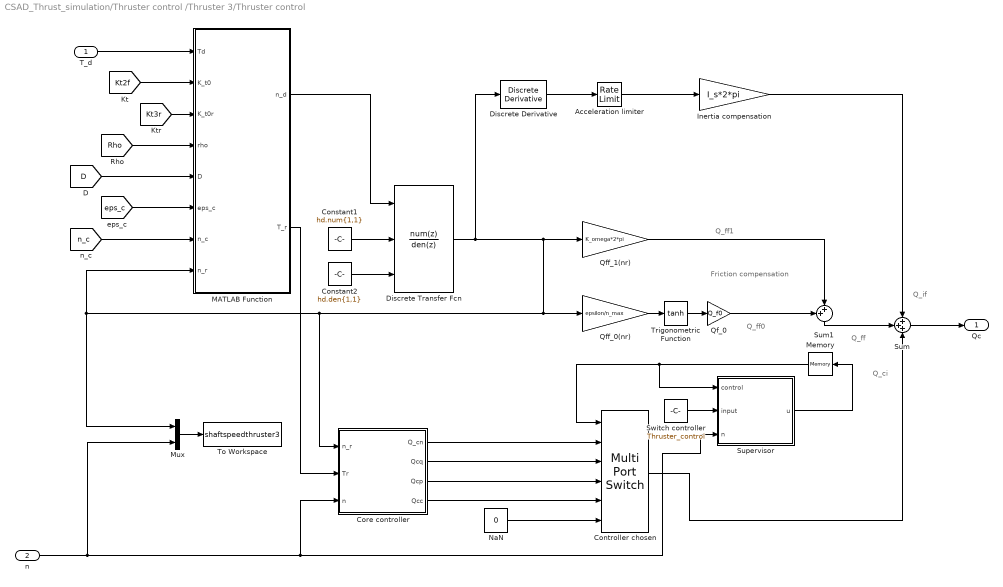
== system CSAD_Thrust_simulation/Thruster control /Thruster 3/Thruster control ==
  note: Q_ci
  note: Q_if
  note: Q_ff
  note: Q_ff0
  note: Q_ff1
  note: Friction compensation
  "T_d " : Inport
  n : Inport  Port=2
  Acceleration limiter : RateLimiter  RisingSlewLimit=Max_Acceleration  FallingSlewLimit=-Max_Acceleration  SampleTimeMode=inherited
  Constant1 : Constant  Value=hd.num{1,1}  VectorParams1D=off
  Constant2 : Constant  Value=hd.den{1,1}  VectorParams1D=off
  Controller chosen : MultiPortSwitch  Inputs=5
  Core controller : Subsystem
  Discrete Transfer Fcn : DiscreteTransferFcn  NumeratorSource=Input port  Numerator=[8.76e-05 0.0003481 8.648e-05]  DenominatorSource=Input port  Denominator=[1 -1.974 0.9746]  SampleTime=0.01  a0EqualsOne=on
      settings: InputPortMap=u0,p1,p3
  Discrete Derivative : simulink/Discrete/Discrete Derivative  gainval=1.0  ICPrevScaledInput=0.0  InputProcessing=Inherited  OutMin=[]  OutMax=[]  OutDataType=fixdt(1, 16)  OutScaling=2^-10  DoSatur=off
  Inertia compensation : Gain  Gain=I_s*2*pi
  MATLAB Function : MATLAB Function  TreatAsAtomicUnit=on
  Memory : Memory  X0=1
  Mux : Mux  Inputs=2
  NaN : Constant  Value=0
  Qf_0 : Gain  Gain=Q_f0
  Qff_0(nr) : Gain  Gain=epsilon/n_max
  Qff_1(nr) : Gain  Gain=K_omega*2*pi
  Sum : Sum  Inputs=+++
  Sum1 : Sum  Inputs=++|
  Supervisor : MATLAB Function  TreatAsAtomicUnit=on
  Switch controller : Constant  Value=Thruster_control
  To Workspace : ToWorkspace  VariableName=shaftspeedthruster3  SaveFormat=Timeseries  SampleTime=-1
  Trigonometric Function : Trigonometry  Operator=tanh
  Qc : Outport
  wires:
  MATLAB Function/2(T_r) -> Core controller/2("Tr ")
  Discrete Derivative/1 -> Acceleration limiter/1
  Qff_0(nr)/1 -> Trigonometric Function/1
  Trigonometric Function/1 -> Qf_0/1
  Sum1/1 -> Sum/2
  Core controller/1(Q_cn) -> Controller chosen/2
  Core controller/4(Qcc) -> Controller chosen/5
  NaN/1 -> Controller chosen/6
  Supervisor/1(u) -> Memory/1
  Memory/1 -> Supervisor/1(control), Controller chosen/1
  Qff_1(nr)/1 -> Sum1/2
  Qf_0/1 -> Sum1/1
  Controller chosen/1 -> Sum/3
  Inertia compensation/1 -> Sum/1
  Core controller/3(Qcp) -> Controller chosen/4
  Core controller/2(Qcq) -> Controller chosen/3
  Switch controller/1 -> Supervisor/2(input)
  "T_d "/1 -> MATLAB Function/1(Td)
  [Rho] -> MATLAB Function/4(rho)
  [D] -> MATLAB Function/5(D)
  [eps_c] -> MATLAB Function/6(eps_c)
  [n_c] -> MATLAB Function/7(n_c)
  Constant1/1 -> Discrete Transfer Fcn/2
  Constant2/1 -> Discrete Transfer Fcn/3
  MATLAB Function/1(n_d) -> Discrete Transfer Fcn/1
  n/1 -> Mux/2, Core controller/3("n "), Supervisor/3(n)
  Mux/1 -> To Workspace/1
  Acceleration limiter/1 -> Inertia compensation/1
  Discrete Transfer Fcn/1 -> Discrete Derivative/1, MATLAB Function/8(n_r), Mux/1, Core controller/1(n_r), Qff_0(nr)/1, Qff_1(nr)/1
  Sum/1 -> Qc/1
  [Kt2f] -> MATLAB Function/2(K_t0)
  [Kt3r] -> MATLAB Function/3(K_t0r)

== system CSAD_Thrust_simulation/Thruster control /Thruster 4/Propeller Hydrodynamics ==
  env : Inport
  n : Inport  Port=2
  Actual Force and Torque : MATLAB Function  TreatAsAtomicUnit=on
  Ta : Outport
  Qa : Outport  Port=2
  wires:
  n/1 -> Actual Force and Torque/1(n)
  [D] -> Actual Force and Torque/7(D)
  [Kq4f] -> Actual Force and Torque/2(Kq)
  Actual Force and Torque/2(Qa) -> Qa/1
  [Rho] -> Actual Force and Torque/6(Rho)
  env/1 -> Actual Force and Torque/9(env)
  [Kt4f] -> Actual Force and Torque/3(Kt)
  Actual Force and Torque/1(Ta) -> Ta/1
  [Kt4r] -> Actual Force and Torque/4(Ktr)
  [Kq4r] -> Actual Force and Torque/5(Kqr)
  [eps_c] -> Actual Force and Torque/8(eps_c)

== system CSAD_Thrust_simulation/Thruster control /Thruster 4/Shaft dynamics ==
  Qm : Inport
  Qa : Inport  Port=2
  Constant : Constant  Value=0
  Finding rotation speed : Gain  Gain=1/(2*pi*I_s)
  Integrator : Integrator  ExternalReset=either
  K_omega : Gain  Gain=K_omega*2*pi
  Sum : Sum  Inputs=-+-
  n : Outport
  wires:
  Qm/1 -> Sum/2
  Sum/1 -> Finding rotation speed/1
  Qa/1 -> Sum/1
  K_omega/1 -> Sum/3
  Finding rotation speed/1 -> Integrator/1
  Integrator/1 -> K_omega/1, n/1
  Constant/1 -> Integrator/2

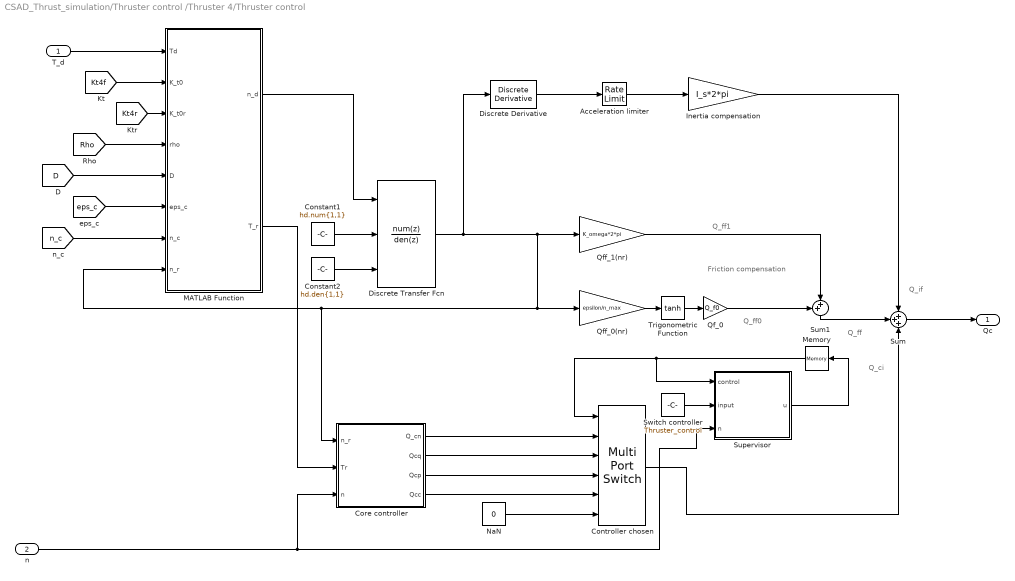
== system CSAD_Thrust_simulation/Thruster control /Thruster 4/Thruster control ==
  note: Q_ci
  note: Q_if
  note: Q_ff
  note: Q_ff0
  note: Q_ff1
  note: Friction compensation
  "T_d " : Inport
  n : Inport  Port=2
  Acceleration limiter : RateLimiter  RisingSlewLimit=Max_Acceleration  FallingSlewLimit=-Max_Acceleration  SampleTimeMode=inherited
  Constant1 : Constant  Value=hd.num{1,1}  VectorParams1D=off
  Constant2 : Constant  Value=hd.den{1,1}  VectorParams1D=off
  Controller chosen : MultiPortSwitch  Inputs=5
  Core controller : Subsystem
  Discrete Transfer Fcn : DiscreteTransferFcn  NumeratorSource=Input port  Numerator=[8.76e-05 0.0003481 8.648e-05]  DenominatorSource=Input port  Denominator=[1 -1.974 0.9746]  SampleTime=0.01  a0EqualsOne=on
      settings: InputPortMap=u0,p1,p3
  Discrete Derivative : simulink/Discrete/Discrete Derivative  gainval=1.0  ICPrevScaledInput=0.0  InputProcessing=Inherited  OutMin=[]  OutMax=[]  OutDataType=fixdt(1, 16)  OutScaling=2^-10  DoSatur=off
  Inertia compensation : Gain  Gain=I_s*2*pi
  MATLAB Function : MATLAB Function  TreatAsAtomicUnit=on
  Memory : Memory  X0=1
  NaN : Constant  Value=0
  Qf_0 : Gain  Gain=Q_f0
  Qff_0(nr) : Gain  Gain=epsilon/n_max
  Qff_1(nr) : Gain  Gain=K_omega*2*pi
  Sum : Sum  Inputs=+++
  Sum1 : Sum  Inputs=++|
  Supervisor : MATLAB Function  TreatAsAtomicUnit=on
  Switch controller : Constant  Value=Thruster_control
  Trigonometric Function : Trigonometry  Operator=tanh
  Qc : Outport
  wires:
  MATLAB Function/2(T_r) -> Core controller/2("Tr ")
  Discrete Derivative/1 -> Acceleration limiter/1
  Qff_0(nr)/1 -> Trigonometric Function/1
  Trigonometric Function/1 -> Qf_0/1
  Sum1/1 -> Sum/2
  Core controller/1(Q_cn) -> Controller chosen/2
  Core controller/4(Qcc) -> Controller chosen/5
  NaN/1 -> Controller chosen/6
  Supervisor/1(u) -> Memory/1
  Memory/1 -> Supervisor/1(control), Controller chosen/1
  Qff_1(nr)/1 -> Sum1/2
  Qf_0/1 -> Sum1/1
  Controller chosen/1 -> Sum/3
  Inertia compensation/1 -> Sum/1
  Core controller/3(Qcp) -> Controller chosen/4
  Core controller/2(Qcq) -> Controller chosen/3
  Switch controller/1 -> Supervisor/2(input)
  "T_d "/1 -> MATLAB Function/1(Td)
  [Rho] -> MATLAB Function/4(rho)
  [D] -> MATLAB Function/5(D)
  [eps_c] -> MATLAB Function/6(eps_c)
  [n_c] -> MATLAB Function/7(n_c)
  Constant1/1 -> Discrete Transfer Fcn/2
  Constant2/1 -> Discrete Transfer Fcn/3
  MATLAB Function/1(n_d) -> Discrete Transfer Fcn/1
  n/1 -> Supervisor/3(n), Core controller/3("n ")
  Acceleration limiter/1 -> Inertia compensation/1
  Discrete Transfer Fcn/1 -> Discrete Derivative/1, MATLAB Function/8(n_r), Core controller/1(n_r), Qff_0(nr)/1, Qff_1(nr)/1
  Sum/1 -> Qc/1
  [Kt4f] -> MATLAB Function/2(K_t0)
  [Kt4r] -> MATLAB Function/3(K_t0r)

== system CSAD_Thrust_simulation/Thruster control /Thruster 5/Propeller Hydrodynamics ==
  env : Inport
  n : Inport  Port=2
  Actual Force and Torque : MATLAB Function  TreatAsAtomicUnit=on
  Ta : Outport
  Qa : Outport  Port=2
  wires:
  n/1 -> Actual Force and Torque/1(n)
  [D] -> Actual Force and Torque/7(D)
  [Kq5f] -> Actual Force and Torque/2(Kq)
  Actual Force and Torque/2(Qa) -> Qa/1
  [Rho] -> Actual Force and Torque/6(Rho)
  env/1 -> Actual Force and Torque/9(env)
  [Kt5f] -> Actual Force and Torque/3(Kt)
  Actual Force and Torque/1(Ta) -> Ta/1
  [Kt5r] -> Actual Force and Torque/4(Ktr)
  [Kq5r] -> Actual Force and Torque/5(Kqr)
  [eps_c] -> Actual Force and Torque/8(eps_c)

== system CSAD_Thrust_simulation/Thruster control /Thruster 5/Shaft dynamics ==
  Qm : Inport
  Qa : Inport  Port=2
  Constant : Constant  Value=0
  Finding rotation speed : Gain  Gain=1/(2*pi*I_s)
  Integrator : Integrator  ExternalReset=either
  K_omega : Gain  Gain=K_omega*2*pi
  Sum : Sum  Inputs=-+-
  n : Outport
  wires:
  Qm/1 -> Sum/2
  Sum/1 -> Finding rotation speed/1
  Qa/1 -> Sum/1
  K_omega/1 -> Sum/3
  Finding rotation speed/1 -> Integrator/1
  Integrator/1 -> K_omega/1, n/1
  Constant/1 -> Integrator/2

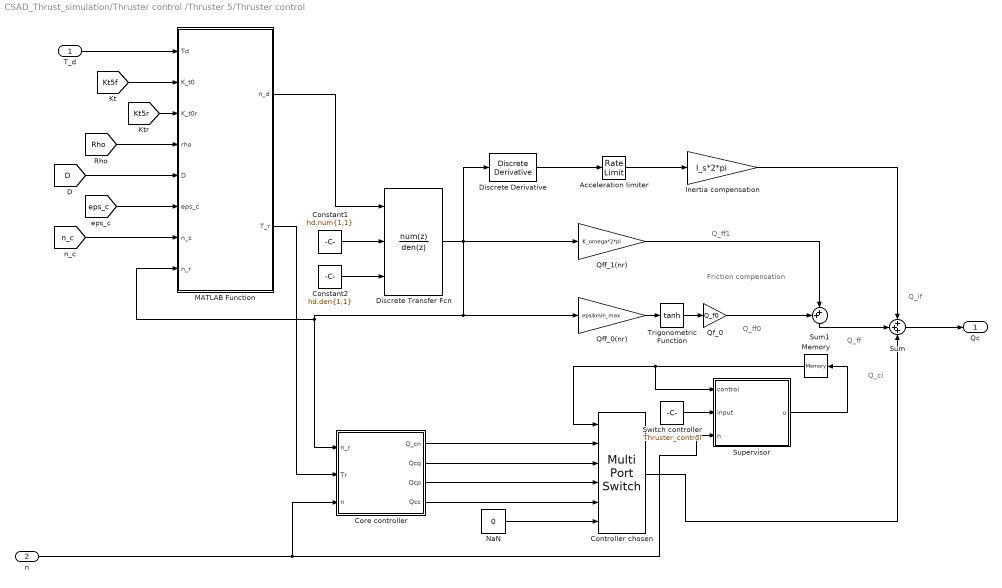
== system CSAD_Thrust_simulation/Thruster control /Thruster 5/Thruster control ==
  note: Q_ci
  note: Q_if
  note: Q_ff
  note: Q_ff0
  note: Q_ff1
  note: Friction compensation
  "T_d " : Inport
  n : Inport  Port=2
  Acceleration limiter : RateLimiter  RisingSlewLimit=Max_Acceleration  FallingSlewLimit=-Max_Acceleration  SampleTimeMode=inherited
  Constant1 : Constant  Value=hd.num{1,1}  VectorParams1D=off
  Constant2 : Constant  Value=hd.den{1,1}  VectorParams1D=off
  Controller chosen : MultiPortSwitch  Inputs=5
  Core controller : Subsystem
  Discrete Transfer Fcn : DiscreteTransferFcn  NumeratorSource=Input port  Numerator=[8.76e-05 0.0003481 8.648e-05]  DenominatorSource=Input port  Denominator=[1 -1.974 0.9746]  SampleTime=0.01  a0EqualsOne=on
      settings: InputPortMap=u0,p1,p3
  Discrete Derivative : simulink/Discrete/Discrete Derivative  gainval=1.0  ICPrevScaledInput=0.0  InputProcessing=Inherited  OutMin=[]  OutMax=[]  OutDataType=fixdt(1, 16)  OutScaling=2^-10  DoSatur=off
  Inertia compensation : Gain  Gain=I_s*2*pi
  MATLAB Function : MATLAB Function  TreatAsAtomicUnit=on
  Memory : Memory  X0=1
  NaN : Constant  Value=0
  Qf_0 : Gain  Gain=Q_f0
  Qff_0(nr) : Gain  Gain=epsilon/n_max
  Qff_1(nr) : Gain  Gain=K_omega*2*pi
  Sum : Sum  Inputs=+++
  Sum1 : Sum  Inputs=++|
  Supervisor : MATLAB Function  TreatAsAtomicUnit=on
  Switch controller : Constant  Value=Thruster_control
  Trigonometric Function : Trigonometry  Operator=tanh
  Qc : Outport
  wires:
  MATLAB Function/2(T_r) -> Core controller/2("Tr ")
  Discrete Derivative/1 -> Acceleration limiter/1
  Qff_0(nr)/1 -> Trigonometric Function/1
  Trigonometric Function/1 -> Qf_0/1
  Sum1/1 -> Sum/2
  Core controller/1(Q_cn) -> Controller chosen/2
  Core controller/4(Qcc) -> Controller chosen/5
  NaN/1 -> Controller chosen/6
  Supervisor/1(u) -> Memory/1
  Memory/1 -> Supervisor/1(control), Controller chosen/1
  Qff_1(nr)/1 -> Sum1/2
  Qf_0/1 -> Sum1/1
  Controller chosen/1 -> Sum/3
  Inertia compensation/1 -> Sum/1
  Core controller/3(Qcp) -> Controller chosen/4
  Core controller/2(Qcq) -> Controller chosen/3
  Switch controller/1 -> Supervisor/2(input)
  [Rho] -> MATLAB Function/4(rho)
  [D] -> MATLAB Function/5(D)
  [eps_c] -> MATLAB Function/6(eps_c)
  [n_c] -> MATLAB Function/7(n_c)
  Constant1/1 -> Discrete Transfer Fcn/2
  Constant2/1 -> Discrete Transfer Fcn/3
  MATLAB Function/1(n_d) -> Discrete Transfer Fcn/1
  n/1 -> Supervisor/3(n), Core controller/3("n ")
  Acceleration limiter/1 -> Inertia compensation/1
  Discrete Transfer Fcn/1 -> Discrete Derivative/1, Qff_0(nr)/1, Core controller/1(n_r), MATLAB Function/8(n_r), Qff_1(nr)/1
  Sum/1 -> Qc/1
  "T_d "/1 -> MATLAB Function/1(Td)
  [Kt5f] -> MATLAB Function/2(K_t0)
  [Kt5r] -> MATLAB Function/3(K_t0r)

== system CSAD_Thrust_simulation/Thruster control /Thruster 6/Propeller Hydrodynamics ==
  env : Inport
  n : Inport  Port=2
  Actual Force and Torque : MATLAB Function  TreatAsAtomicUnit=on
  Ta : Outport
  Qa : Outport  Port=2
  wires:
  n/1 -> Actual Force and Torque/1(n)
  [D] -> Actual Force and Torque/7(D)
  [Kq6f] -> Actual Force and Torque/2(Kq)
  Actual Force and Torque/2(Qa) -> Qa/1
  [Rho] -> Actual Force and Torque/6(Rho)
  env/1 -> Actual Force and Torque/9(env)
  [Kt6f] -> Actual Force and Torque/3(Kt)
  Actual Force and Torque/1(Ta) -> Ta/1
  [Kt6r] -> Actual Force and Torque/4(Ktr)
  [Kq6r] -> Actual Force and Torque/5(Kqr)
  [eps_c] -> Actual Force and Torque/8(eps_c)

== system CSAD_Thrust_simulation/Thruster control /Thruster 6/Shaft dynamics ==
  Qm : Inport
  Qa : Inport  Port=2
  Constant : Constant  Value=0
  Finding rotation speed : Gain  Gain=1/(2*pi*I_s)
  Integrator : Integrator  ExternalReset=either
  K_omega : Gain  Gain=K_omega*2*pi
  Sum : Sum  Inputs=-+-
  n : Outport
  wires:
  Qm/1 -> Sum/2
  Sum/1 -> Finding rotation speed/1
  Qa/1 -> Sum/1
  K_omega/1 -> Sum/3
  Finding rotation speed/1 -> Integrator/1
  Integrator/1 -> K_omega/1, n/1
  Constant/1 -> Integrator/2

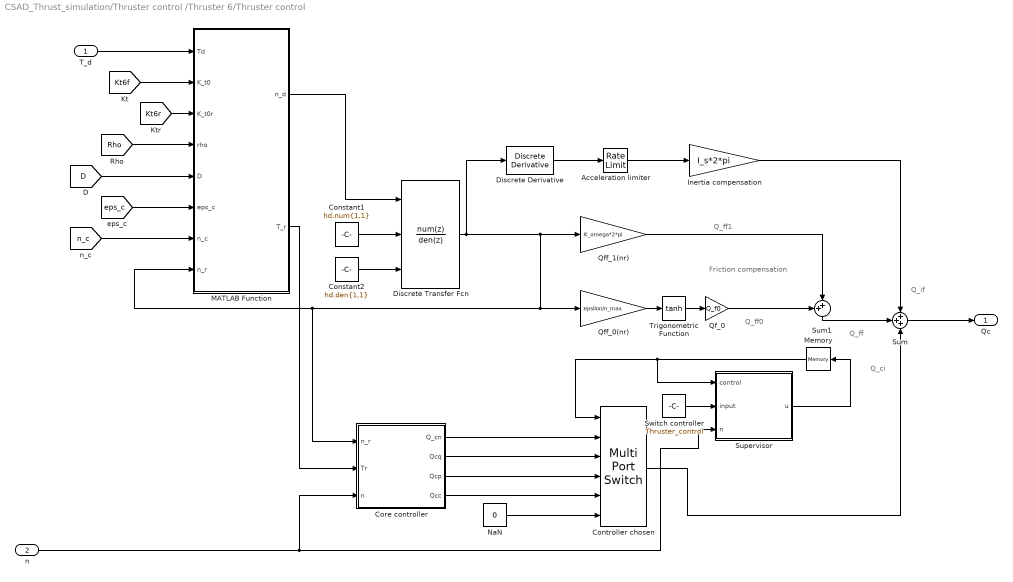
== system CSAD_Thrust_simulation/Thruster control /Thruster 6/Thruster control ==
  note: Q_ci
  note: Q_if
  note: Q_ff
  note: Q_ff0
  note: Q_ff1
  note: Friction compensation
  "T_d " : Inport
  n : Inport  Port=2
  Acceleration limiter : RateLimiter  RisingSlewLimit=Max_Acceleration  FallingSlewLimit=-Max_Acceleration  SampleTimeMode=inherited
  Constant1 : Constant  Value=hd.num{1,1}  VectorParams1D=off
  Constant2 : Constant  Value=hd.den{1,1}  VectorParams1D=off
  Controller chosen : MultiPortSwitch  Inputs=5
  Core controller : Subsystem
  Discrete Transfer Fcn : DiscreteTransferFcn  NumeratorSource=Input port  Numerator=[8.76e-05 0.0003481 8.648e-05]  DenominatorSource=Input port  Denominator=[1 -1.974 0.9746]  SampleTime=0.01  a0EqualsOne=on
      settings: InputPortMap=u0,p1,p3
  Discrete Derivative : simulink/Discrete/Discrete Derivative  gainval=1.0  ICPrevScaledInput=0.0  InputProcessing=Inherited  OutMin=[]  OutMax=[]  OutDataType=fixdt(1, 16)  OutScaling=2^-10  DoSatur=off
  Inertia compensation : Gain  Gain=I_s*2*pi
  MATLAB Function : MATLAB Function  TreatAsAtomicUnit=on
  Memory : Memory  X0=1
  NaN : Constant  Value=0
  Qf_0 : Gain  Gain=Q_f0
  Qff_0(nr) : Gain  Gain=epsilon/n_max
  Qff_1(nr) : Gain  Gain=K_omega*2*pi
  Sum : Sum  Inputs=+++
  Sum1 : Sum  Inputs=++|
  Supervisor : MATLAB Function  TreatAsAtomicUnit=on
  Switch controller : Constant  Value=Thruster_control
  Trigonometric Function : Trigonometry  Operator=tanh
  Qc : Outport
  wires:
  MATLAB Function/2(T_r) -> Core controller/2("Tr ")
  Discrete Derivative/1 -> Acceleration limiter/1
  Qff_0(nr)/1 -> Trigonometric Function/1
  Trigonometric Function/1 -> Qf_0/1
  Sum1/1 -> Sum/2
  Core controller/1(Q_cn) -> Controller chosen/2
  Core controller/4(Qcc) -> Controller chosen/5
  NaN/1 -> Controller chosen/6
  Supervisor/1(u) -> Memory/1
  Memory/1 -> Supervisor/1(control), Controller chosen/1
  Qff_1(nr)/1 -> Sum1/2
  Qf_0/1 -> Sum1/1
  Controller chosen/1 -> Sum/3
  Inertia compensation/1 -> Sum/1
  Core controller/3(Qcp) -> Controller chosen/4
  Core controller/2(Qcq) -> Controller chosen/3
  Switch controller/1 -> Supervisor/2(input)
  [Rho] -> MATLAB Function/4(rho)
  [D] -> MATLAB Function/5(D)
  [eps_c] -> MATLAB Function/6(eps_c)
  [n_c] -> MATLAB Function/7(n_c)
  Constant1/1 -> Discrete Transfer Fcn/2
  Constant2/1 -> Discrete Transfer Fcn/3
  MATLAB Function/1(n_d) -> Discrete Transfer Fcn/1
  n/1 -> Supervisor/3(n), Core controller/3("n ")
  Acceleration limiter/1 -> Inertia compensation/1
  Discrete Transfer Fcn/1 -> Discrete Derivative/1, MATLAB Function/8(n_r), Core controller/1(n_r), Qff_0(nr)/1, Qff_1(nr)/1
  Sum/1 -> Qc/1
  "T_d "/1 -> MATLAB Function/1(Td)
  [Kt6f] -> MATLAB Function/2(K_t0)
  [Kt6r] -> MATLAB Function/3(K_t0r)

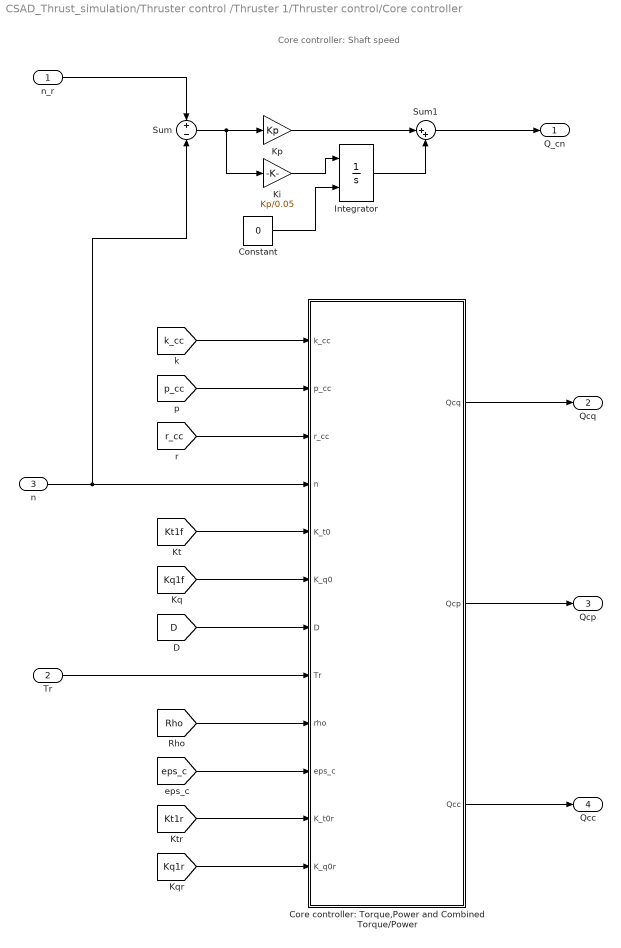
== system CSAD_Thrust_simulation/Thruster control /Thruster 1/Thruster control/Core controller ==
  note: Core controller: Shaft speed
  n_r : Inport
  "Tr " : Inport  Port=2
  "n " : Inport  Port=3
  Constant : Constant  Value=0
  Core controller: Torque,Power and Combined Torque/Power : MATLAB Function  TreatAsAtomicUnit=on
  Integrator : Integrator  ExternalReset=either
  Ki : Gain  Gain=Kp/0.05
  Kp : Gain  Gain=Kp
  Sum : Sum  Inputs=+|-
  Sum1 : Sum  Inputs=|++
  Q_cn : Outport
  Qcq : Outport  Port=2
  Qcp : Outport  Port=3
  Qcc : Outport  Port=4
  wires:
  [k_cc] -> Core controller: Torque,Power and Combined Torque/Power/1(k_cc)
  [p_cc] -> Core controller: Torque,Power and Combined Torque/Power/2(p_cc)
  [r_cc] -> Core controller: Torque,Power and Combined Torque/Power/3(r_cc)
  Core controller: Torque,Power and Combined Torque/Power/3(Qcc) -> Qcc/1
  [Kt1f] -> Core controller: Torque,Power and Combined Torque/Power/5(K_t0)
  [D] -> Core controller: Torque,Power and Combined Torque/Power/7(D)
  [Rho] -> Core controller: Torque,Power and Combined Torque/Power/9(rho)
  "n "/1 -> Sum/2, Core controller: Torque,Power and Combined Torque/Power/4(n)
  "Tr "/1 -> Core controller: Torque,Power and Combined Torque/Power/8(Tr)
  Core controller: Torque,Power and Combined Torque/Power/2(Qcp) -> Qcp/1
  Core controller: Torque,Power and Combined Torque/Power/1(Qcq) -> Qcq/1
  n_r/1 -> Sum/1
  Ki/1 -> Integrator/1
  Kp/1 -> Sum1/1
  Integrator/1 -> Sum1/2
  Sum1/1 -> Q_cn/1
  Sum/1 -> Ki/1, Kp/1
  Constant/1 -> Integrator/2
  [eps_c] -> Core controller: Torque,Power and Combined Torque/Power/10(eps_c)
  [Kt1r] -> Core controller: Torque,Power and Combined Torque/Power/11(K_t0r)
  [Kq1f] -> Core controller: Torque,Power and Combined Torque/Power/6(K_q0)
  [Kq1r] -> Core controller: Torque,Power and Combined Torque/Power/12(K_q0r)

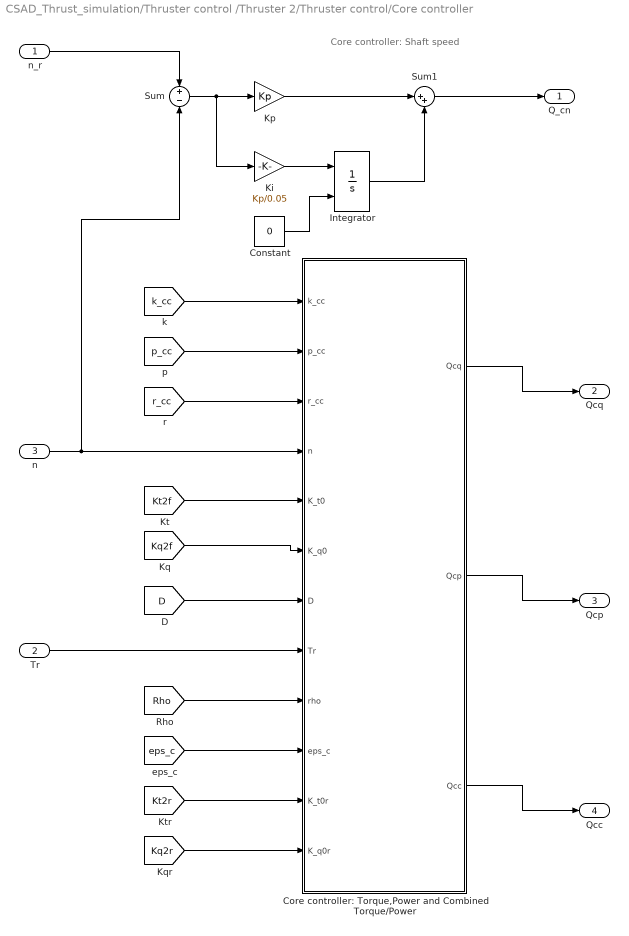
== system CSAD_Thrust_simulation/Thruster control /Thruster 2/Thruster control/Core controller ==
  note: Core controller: Shaft speed
  n_r : Inport
  "Tr " : Inport  Port=2
  "n " : Inport  Port=3
  Constant : Constant  Value=0
  Core controller: Torque,Power and Combined Torque/Power : MATLAB Function  TreatAsAtomicUnit=on
  Integrator : Integrator  ExternalReset=either
  Ki : Gain  Gain=Kp/0.05
  Kp : Gain  Gain=Kp
  Sum : Sum  Inputs=+|-
  Sum1 : Sum  Inputs=|++
  Q_cn : Outport
  Qcq : Outport  Port=2
  Qcp : Outport  Port=3
  Qcc : Outport  Port=4
  wires:
  n_r/1 -> Sum/1
  Ki/1 -> Integrator/1
  Kp/1 -> Sum1/1
  Integrator/1 -> Sum1/2
  Sum/1 -> Ki/1, Kp/1
  Sum1/1 -> Q_cn/1
  Constant/1 -> Integrator/2
  [k_cc] -> Core controller: Torque,Power and Combined Torque/Power/1(k_cc)
  [p_cc] -> Core controller: Torque,Power and Combined Torque/Power/2(p_cc)
  [r_cc] -> Core controller: Torque,Power and Combined Torque/Power/3(r_cc)
  Core controller: Torque,Power and Combined Torque/Power/3(Qcc) -> Qcc/1
  [Kt2f] -> Core controller: Torque,Power and Combined Torque/Power/5(K_t0)
  [D] -> Core controller: Torque,Power and Combined Torque/Power/7(D)
  [Kq2f] -> Core controller: Torque,Power and Combined Torque/Power/6(K_q0)
  [Rho] -> Core controller: Torque,Power and Combined Torque/Power/9(rho)
  "n "/1 -> Core controller: Torque,Power and Combined Torque/Power/4(n), Sum/2
  "Tr "/1 -> Core controller: Torque,Power and Combined Torque/Power/8(Tr)
  Core controller: Torque,Power and Combined Torque/Power/2(Qcp) -> Qcp/1
  Core controller: Torque,Power and Combined Torque/Power/1(Qcq) -> Qcq/1
  [eps_c] -> Core controller: Torque,Power and Combined Torque/Power/10(eps_c)
  [Kt2r] -> Core controller: Torque,Power and Combined Torque/Power/11(K_t0r)
  [Kq2r] -> Core controller: Torque,Power and Combined Torque/Power/12(K_q0r)

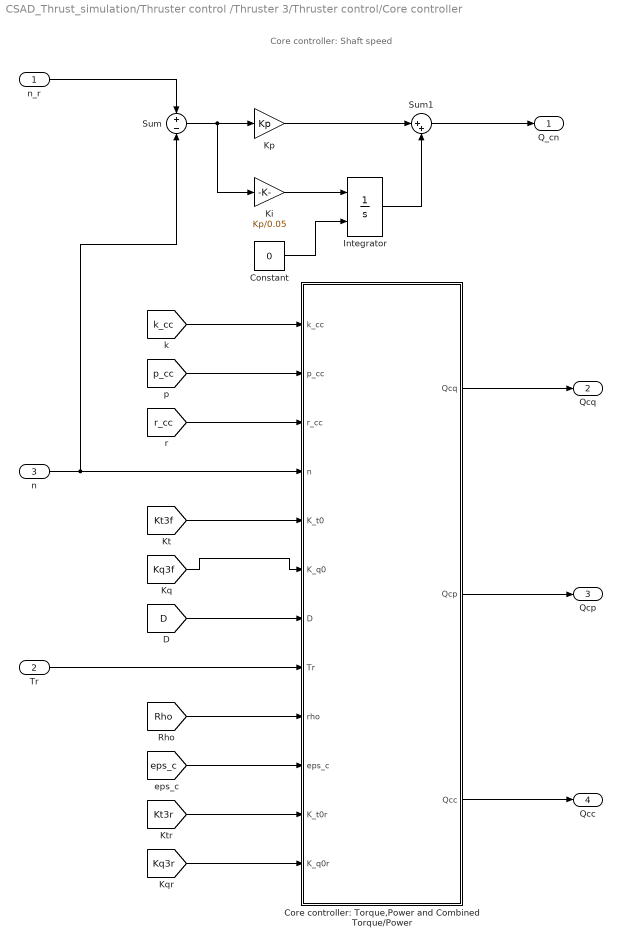
== system CSAD_Thrust_simulation/Thruster control /Thruster 3/Thruster control/Core controller ==
  note: Core controller: Shaft speed
  n_r : Inport
  "Tr " : Inport  Port=2
  "n " : Inport  Port=3
  Constant : Constant  Value=0
  Core controller: Torque,Power and Combined Torque/Power : MATLAB Function  TreatAsAtomicUnit=on
  Integrator : Integrator  ExternalReset=either
  Ki : Gain  Gain=Kp/0.05
  Kp : Gain  Gain=Kp
  Sum : Sum  Inputs=+|-
  Sum1 : Sum  Inputs=|++
  Q_cn : Outport
  Qcq : Outport  Port=2
  Qcp : Outport  Port=3
  Qcc : Outport  Port=4
  wires:
  n_r/1 -> Sum/1
  Ki/1 -> Integrator/1
  Kp/1 -> Sum1/1
  Integrator/1 -> Sum1/2
  Sum/1 -> Ki/1, Kp/1
  Sum1/1 -> Q_cn/1
  Constant/1 -> Integrator/2
  [k_cc] -> Core controller: Torque,Power and Combined Torque/Power/1(k_cc)
  [p_cc] -> Core controller: Torque,Power and Combined Torque/Power/2(p_cc)
  [r_cc] -> Core controller: Torque,Power and Combined Torque/Power/3(r_cc)
  Core controller: Torque,Power and Combined Torque/Power/3(Qcc) -> Qcc/1
  [Kt3f] -> Core controller: Torque,Power and Combined Torque/Power/5(K_t0)
  [D] -> Core controller: Torque,Power and Combined Torque/Power/7(D)
  [Kq3f] -> Core controller: Torque,Power and Combined Torque/Power/6(K_q0)
  [Rho] -> Core controller: Torque,Power and Combined Torque/Power/9(rho)
  "n "/1 -> Sum/2, Core controller: Torque,Power and Combined Torque/Power/4(n)
  "Tr "/1 -> Core controller: Torque,Power and Combined Torque/Power/8(Tr)
  Core controller: Torque,Power and Combined Torque/Power/2(Qcp) -> Qcp/1
  Core controller: Torque,Power and Combined Torque/Power/1(Qcq) -> Qcq/1
  [eps_c] -> Core controller: Torque,Power and Combined Torque/Power/10(eps_c)
  [Kt3r] -> Core controller: Torque,Power and Combined Torque/Power/11(K_t0r)
  [Kq3r] -> Core controller: Torque,Power and Combined Torque/Power/12(K_q0r)
